simulink model "chap5_5sim"  (Simulink 3.00)
settings: Solver=ode45  StartTime=0.0  StopTime=5  RelTol=1e-3
settings Model: LastModifiedBy=liu

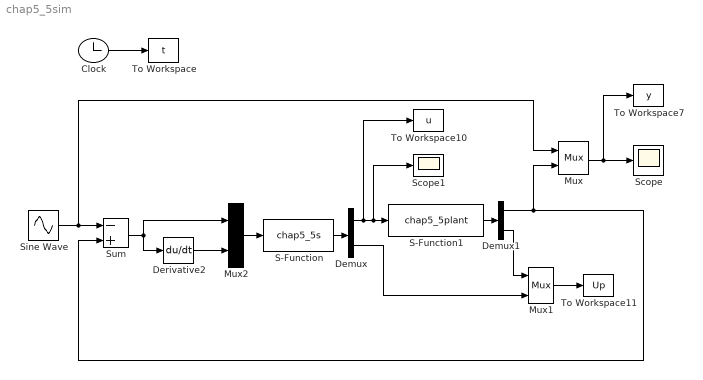
== system chap5_5sim ==
  Clock : Clock
  Demux : Demux  Outputs=2
  Demux1 : Demux  Outputs=2
  Derivative2 : Derivative
  Mux : Mux  Inputs=2
      settings: DisplayOption=none
  Mux1 : Mux  Inputs=2
      settings: DisplayOption=none
  Mux2 : Mux  Inputs=2
      settings: DisplayOption=none
  S-Function : S-Function  FunctionName=chap5_5s  PortCounts=[]  SFunctionModules=''
  S-Function1 : S-Function  FunctionName=chap5_5plant  PortCounts=[]  SFunctionModules=''
  Scope : Scope
      settings: TimeRange=3  YMin=-1  YMax=1  SaveToWorkspace=off  SaveName=ScopeData  MaxRows=500000
  Scope1 : Scope
      settings: TimeRange=5  YMin=-1.25  YMax=0.75  SaveToWorkspace=off  SaveName=ScopeData  MaxRows=500000
  Sine Wave : Sin  Amplitude=1  Frequency=pi  Phase=0  SampleTime=0
  Sum : Sum  Inputs=-+  SaturateOnIntegerOverflow=on
  To Workspace : ToWorkspace  VariableName=t  SampleTime=-1  SaveFormat=Matrix
  To Workspace10 : ToWorkspace  VariableName=u  SampleTime=-1  SaveFormat=Matrix
  To Workspace11 : ToWorkspace  VariableName=Up  SampleTime=-1  SaveFormat=Matrix
  To Workspace7 : ToWorkspace  VariableName=y  SampleTime=-1  SaveFormat=Matrix
  wires:
  S-Function/1 -> Demux/1
  Demux/1 -> S-Function1/1, Scope1/1, To Workspace10/1
  Mux/1 -> Scope/1, To Workspace7/1
  S-Function1/1 -> Demux1/1
  Mux1/1 -> To Workspace11/1
  Demux1/2 -> Mux1/1
  Demux/2 -> Mux1/2
  Demux1/1 -> Mux/2, Sum/2
  Clock/1 -> To Workspace/1
  Mux2/1 -> S-Function/1
  Sine Wave/1 -> Sum/1, Mux/1
  Derivative2/1 -> Mux2/2
  Sum/1 -> Derivative2/1, Mux2/1
